simulink model "sl_subsys_trigerr2"  (Simulink 7.6)
settings: Solver=ode45  StartTime=0.0  StopTime=10.0  RelTol=1e-3
Description:
  | Example of modeling error - ambiguous execution order
settings Model: Creator=The MathWorks Inc.  CovMetricSettings=d  ExtModeAutoUpdateStatusClock=off
settings OptimizationCC: BlockReduction=off  BooleanDataType=off  InitFltsAndDblsToZero=on
settings DebuggingCC: SaveWithParameterizedLinksMsg=none  SignalResolutionControl=TryResolveAllWithWarning  SolverPrmCheckMsg=none  MultiTaskDSMMsg=warning  MultiTaskCondExecSysMsg=none
settings HardwareCC: TargetUnknown=on
settings SFSimCC: SimParseCustomCode=off
settings RTWCC: IncludeERTFirstTime=on
settings CodeAppCC: CustomSymbolStrFcn=$F$N$M
settings GRTTargetCC: TargetFcnLib=ansi_tfl_tmw.mat

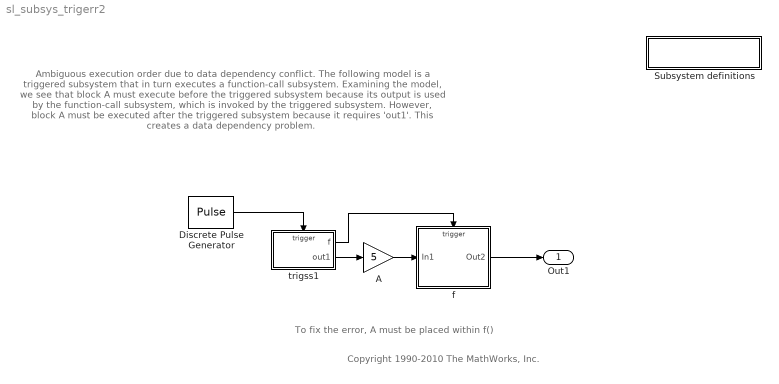
== system sl_subsys_trigerr2 ==
  note: Ambiguous execution order due to data dependency conflict.
      |
      | The following model is a triggered subsystem that in turn
      | executes a function-call subsystem.  Examining the model, we see
      | that block A must execute before the triggered subsystem because
      | its output is used by the function-call subsystem, which is invoked
      | by the triggered subsystem. However, block A must be executed after
      | the triggered subsystem because it requires 'out1'. This creates a
      | data dependency problem.
  note: To fix the error, A must be placed within f()
  note: Copyright 1990-2010 The MathWorks, Inc.
  " Subsystem definitions" : Subsystem
      settings: OpenFcn=helpview([matlabroot,'/toolbox/simulink/simdemos/simfeatures/html/sl_subsys_definitions.html']);
      mask Display: disp('Subsystem\ndefinitions')
  A : Gain  Gain=5  SaturateOnIntegerOverflow=on  OutDataTypeStr=Inherit: Same as input  ParamDataTypeStr=Inherit: Same as input
  Discrete Pulse Generator : DiscretePulseGenerator
  f : Subsystem  TreatAsAtomicUnit=on
  trigss1 : Subsystem  TreatAsAtomicUnit=on
  Out1 : Outport
  wires:
  Discrete Pulse Generator/1 -> trigss1/Trigger
  A/1 -> f/1(In1)
  f/1(Out2) -> Out1/1
  trigss1/1(f) -> f/Trigger
  trigss1/2(out1) -> A/1

== system sl_subsys_trigerr2/ Subsystem definitions ==

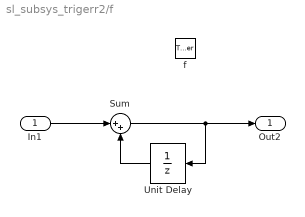
== system sl_subsys_trigerr2/f ==
  In1 : Inport
  f : TriggerPort  TriggerType=function-call
  Sum : Sum  Inputs=|++  SaturateOnIntegerOverflow=on  InputSameDT=on  OutDataTypeStr=Inherit: Same as first input
  Unit Delay : UnitDelay  SampleTime=-1
  Out2 : Outport
  wires:
  Sum/1 -> Unit Delay/1, Out2/1
  Unit Delay/1 -> Sum/2
  In1/1 -> Sum/1

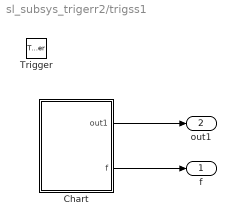
== system sl_subsys_trigerr2/trigss1 ==
  Trigger : TriggerPort
  Chart : Stateflow chart  TreatAsAtomicUnit=on
  f : Outport
  out1 : Outport  Port=2
  wires:
  Chart/1(out1) -> out1/1
  Chart/2(f) -> f/1

== stateflow chart trigss1/Chart ==
  state one/
    entry: f;d2=d2+10;
  state two/
    entry: f;d1 = d1+5;
  one -> two
  two -> one
  (default) -> one
  data: out1 output double; d1 local double; d2 local double
  events: f output FUNCTION_CALL_EVENT
